simulink model "ex_lct_struct"  (R2019a)
settings: Solver=VariableStepAuto  StartTime=0.0  StopTime=10.0  RelTol=1e-3
undefined symbols (not defined in the file or in its folder): structParam
settings Model: Creator=The MathWorks, Inc.  LastModifiedBy=RUOBING
settings DebuggingCC: ArithmeticOperatorsInVariantConditions=warning
settings SFSimCC: SimUseLocalCustomCode=off
settings RTWCC: RTWUseLocalCustomCode=off
settings CodeAppCC: StateflowObjectComments=on

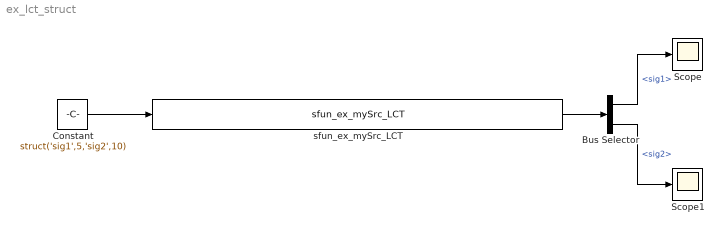
== system ex_lct_struct ==
  Bus Selector : BusSelector  OutputSignals=sig1,sig2
  Constant : Constant  Value=struct('sig1',5,'sig2',10)  OutDataTypeStr=Bus: sigStructType
  Scope : Scope
  Scope1 : Scope
  sfun_ex_mySrc_LCT : S-Function  FunctionName=sfun_ex_mySrc_LCT  Parameters=SParameter1  SFunctionDeploymentMode=off  EnableBusSupport=off  mask(Legacy Function){SFunctionSpec=void myFcn(sigStructType u1[1], paramStructType p1[1], sigStructType y1[1]), SParameter1=structParam, ShowSpec=on}
      mask prompts: SParameter1 "P1:"; ShowSpec "Display function specification"
      mask help:
      | This block allows you to call the legacy functions specified by the following Legacy Code Tool definition:
      | def.SFunctionName = 'sfun_ex_mySrc_LCT';
      | def.OutputFcnSpec = 'void myFcn(sigStructType u1[1], paramStructType p1[1], sigStructType y1[1])';
      | def.HeaderFiles = {'ex_myTypes_LCT.h'};
      mask Help: <p>This block was generated automatically by the Legacy Code Tool. For detailed help on this tool, call<a href="matlab:legacy_code('help')"> legacy_code('help')</a>.</p>
      mask Callback ShowSpec:
      | if strcmp(get_param(gcbh, 'ShowSpec'), 'on')
      |   set_param(gcbh, 'MaskDisplay', sprintf('fprintf(''%s'');', get_param(gcbh, 'SFunctionSpec')));
      | else
      |   set_param(gcbh, 'MaskDisplay', sprintf('fprintf(''%s'');', get_param(gcbh, 'FunctionName')));
      | end
      mask Display: fprintf('void myFcn(sigStructType u1[1], paramStructType p1[1], sigStructType y1[1])');
  wires:
  sfun_ex_mySrc_LCT/1 -> Bus Selector/1
  Constant/1 -> sfun_ex_mySrc_LCT/1
  Bus Selector/1 -> Scope/1  "<sig1>"
  Bus Selector/2 -> Scope1/1  "<sig2>"
